simulink model "slexPowerWindowCntlCoverage"  (R2014b)
settings: Solver=ode23  StartTime=0.0  StopTime=10  FixedStep=1e-4  RelTol=1e-3
libraries: simulink x4
Description:
  | Controller Model Coverage
  | 
  | This model contains the power window controller which is a state machine. This model also
  | contains inputs to the controller which are repeating sequence blocks.
  | 
  | You can use the Simulink Verification and Validation(TM) Model Coverage tool
  | to validate the discrete event control of the window. The Model Coverage tool
  | helps determine the extent to which a model test case exercises the conditional
  | branches of the controller.
settings Model: ModifiedByFormat=The MathWorks Inc.  RecordCoverage=on  CovHTMLOptions=-sRT=1 -sVT=0 -aTS=1 -bRG=1 -bTC=1 -hTR=0 -nFC=0 -scm=1 -bcm=1 -xEv=0  CovModelRefEnable=all  ExtModeAutoUpdateStatusClock=off  Creator=The MathWorks Inc.  LastModifiedBy=The MathWorks Inc.
settings DataIOCC: SignalLoggingName=Logsout
settings OptimizationCC: BooleanDataType=off  ExpressionDepthLimit=2147483647  InitFltsAndDblsToZero=on  AccelVerboseBuild=on
settings DebuggingCC: SaveWithParameterizedLinksMsg=none  UnderspecifiedInitializationDetection=Classic  MergeDetectMultiDrivingBlocksExec=none  SignalResolutionControl=TryResolveAllWithWarning  SolverPrmCheckMsg=none  MultiTaskDSMMsg=warning  MultiTaskCondExecSysMsg=none  FcnCallInpInsideContextMsg=UseLocalSettings  StateNameClashWarn=warning
settings HardwareCC: ProdHWDeviceType=Generic->Unspecified (assume 32-bit Generic)
settings SFSimCC: SimParseCustomCode=off
settings RTWCC: IncludeERTFirstTime=on
settings GRTTargetCC: TargetFcnLib=ansi_tfl_tmw.mat  CombineOutputUpdateFcns=off  GRTInterface=on

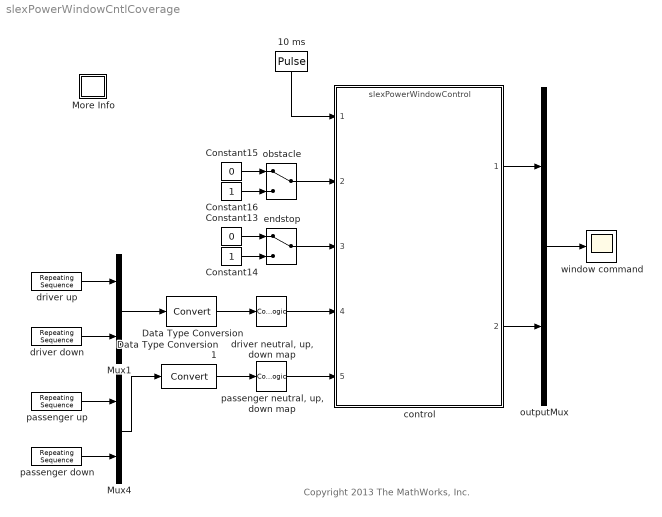
== system slexPowerWindowCntlCoverage ==
  note: Copyright 2013 The MathWorks, Inc.
  10 ms : DiscretePulseGenerator  SampleTime=10e-3
  Constant13 : Constant  Value=0  OutDataTypeStr=boolean
  Constant14 : Constant  OutDataTypeStr=boolean
  Constant15 : Constant  Value=0  OutDataTypeStr=boolean
  Constant16 : Constant  OutDataTypeStr=boolean
  Data Type Conversion : DataTypeConversion
  Data Type Conversion1 : DataTypeConversion
  More Info : Subsystem
      settings: OpenFcn=showdemo('slexPowerWindowScript')
      mask Display: disp('?')
  Mux1 : Mux  Inputs=2
  Mux4 : Mux  Inputs=2
  "control " : ModelReference  ModelNameDialog=slexPowerWindowControl.slx  SimulationMode=Normal  ModelReferenceVersion=1.83  CopyOfModelName=slexPowerWindowControl.slx  DefaultDataLogging=on
  "driver neutral, up, down map" : CombinatorialLogic  TruthTable=[1 0 0;0 0 1;0 1 0;1 0 0]  SampleTime=0.01
  driver down : simulink/Sources/Repeating Sequence  rep_seq_t=[0 1 2 3 4 5 6]  rep_seq_y=[0 1 0 0 1 1 0]
  driver up : simulink/Sources/Repeating Sequence  rep_seq_t=[0 1 2 3 4 5 6]  rep_seq_y=[0 0 1 0 1 0 1]
  endstop : ManualSwitch
  obstacle : ManualSwitch
  outputMux : Mux  Inputs=2
  "passenger neutral, up, down map" : CombinatorialLogic  TruthTable=[1 0 0;0 0 1;0 1 0;1 0 0]  SampleTime=0.01
  passenger down : simulink/Sources/Repeating Sequence  rep_seq_t=[0 1 2 3 4 5 6]  rep_seq_y=[0 0 0 1 0 1 1]
  passenger up : simulink/Sources/Repeating Sequence  rep_seq_t=[0 1 2 3 4 5 6]  rep_seq_y=[0 0 0 0 0 0 0]
  window command : Scope
      settings: YMin=0  YMax=1
  wires:
  passenger down/1 -> Mux4/2
  driver down/1 -> Mux1/2
  Mux4/1 -> Data Type Conversion1/1
  Mux1/1 -> Data Type Conversion/1
  passenger up/1 -> Mux4/1
  driver up/1 -> Mux1/1
  "control "/1 -> outputMux/1
  "control "/2 -> outputMux/2
  outputMux/1 -> window command/1
  Constant13/1 -> endstop/1
  Constant14/1 -> endstop/2
  Constant15/1 -> obstacle/1
  Constant16/1 -> obstacle/2
  Data Type Conversion/1 -> "driver neutral, up, down map"/1
  Data Type Conversion1/1 -> "passenger neutral, up, down map"/1
  "passenger neutral, up, down map"/1 -> "control "/5
  "driver neutral, up, down map"/1 -> "control "/4
  endstop/1 -> "control "/3
  obstacle/1 -> "control "/2
  10 ms/1 -> "control "/1

== system slexPowerWindowCntlCoverage/More Info ==
